simulink model "extra_simulink"  (R2021a)
settings: Solver=VariableStepAuto  StartTime=0.0  StopTime=10  MaxStep=1e-4  RelTol=1e-3
undefined symbols (not defined in the file): b1, b2, b3, F_1, F_2, F_3, k1, k2, k3, m1, m2, m3, time_F_1, time_F_2, time_F_3, x1_0, x2_0, x3_0
settings Model: Creator=SPb19  LastModifiedBy=SPb19

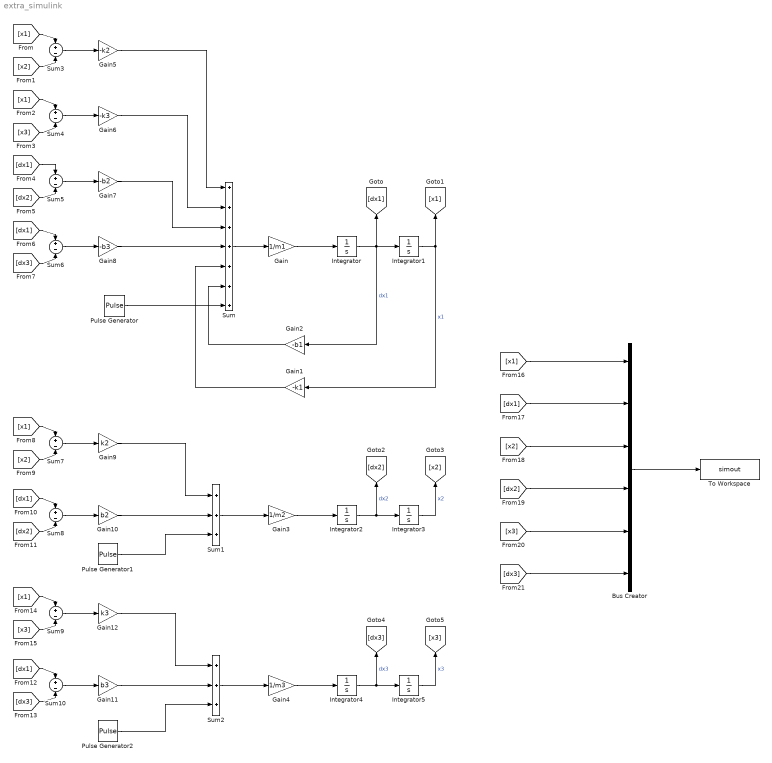
== system extra_simulink ==
  Bus Creator : BusCreator  Inputs=6
  Gain : Gain  Gain=1/m1
  Gain1 : Gain  Gain=-k1
  Gain10 : Gain  Gain=b2
  Gain11 : Gain  Gain=b3
  Gain12 : Gain  Gain=k3
  Gain2 : Gain  Gain=-b1
  Gain3 : Gain  Gain=1/m2
  Gain4 : Gain  Gain=1/m3
  Gain5 : Gain  Gain=-k2
  Gain6 : Gain  Gain=-k3
  Gain7 : Gain  Gain=-b2
  Gain8 : Gain  Gain=-b3
  Gain9 : Gain  Gain=k2
  Integrator : Integrator
  Integrator1 : Integrator  InitialCondition=x1_0
  Integrator2 : Integrator
  Integrator3 : Integrator  InitialCondition=x2_0
  Integrator4 : Integrator
  Integrator5 : Integrator  InitialCondition=x3_0
  Pulse Generator : DiscretePulseGenerator  PulseType=Time based  Amplitude=F_1  Period=t + 10  PulseWidth=100 * time_F_1 / (t + 10)
  Pulse Generator1 : DiscretePulseGenerator  PulseType=Time based  Amplitude=F_2  Period=t + 10  PulseWidth=100 * time_F_2 / (t + 10)
  Pulse Generator2 : DiscretePulseGenerator  PulseType=Time based  Amplitude=F_3  Period=t + 10  PulseWidth=100 * time_F_3 / (t + 10)
  Sum : Sum  Inputs=+++++++
  Sum1 : Sum  Inputs=+++
  Sum{3..10} (8 alike) : Sum  Inputs=+-
  Sum2 : Sum  Inputs=+++
  To Workspace : ToWorkspace  VariableName=simout  SaveFormat=Timeseries  SampleTime=-1
  wires:
  Gain/1 -> Integrator/1
  Integrator/1 -> [dx1], Gain2/1, Integrator1/1  "dx1"
  Sum/1 -> Gain/1
  Integrator1/1 -> [x1], Gain1/1  "x1"
  Gain1/1 -> Sum/5
  Gain2/1 -> Sum/6
  Sum1/1 -> Gain3/1
  Integrator3/1 -> [x2]  "x2"
  Integrator2/1 -> [dx2], Integrator3/1  "dx2"
  Gain3/1 -> Integrator2/1
  Integrator4/1 -> [dx3], Integrator5/1  "dx3"
  Gain4/1 -> Integrator4/1
  Integrator5/1 -> [x3]  "x3"
  Sum2/1 -> Gain4/1
  [x1] -> Sum3/1
  [x2] -> Sum3/2
  Sum3/1 -> Gain5/1
  Gain5/1 -> Sum/1
  Sum4/1 -> Gain6/1
  [x1] -> Sum4/1
  [x3] -> Sum4/2
  Gain6/1 -> Sum/2
  [dx2] -> Sum5/2
  [dx1] -> Sum5/1
  Sum5/1 -> Gain7/1
  Gain7/1 -> Sum/3
  Sum6/1 -> Gain8/1
  [dx1] -> Sum6/1
  [dx3] -> Sum6/2
  Gain8/1 -> Sum/4
  Sum7/1 -> Gain9/1
  [x1] -> Sum7/1
  [x2] -> Sum7/2
  Gain9/1 -> Sum1/1
  Sum8/1 -> Gain10/1
  [dx1] -> Sum8/1
  [dx2] -> Sum8/2
  Gain10/1 -> Sum1/2
  [x3] -> Sum9/2
  [dx3] -> Sum10/2
  [dx1] -> Sum10/1
  Sum10/1 -> Gain11/1
  Sum9/1 -> Gain12/1
  [x1] -> Sum9/1
  Gain12/1 -> Sum2/1
  Gain11/1 -> Sum2/2
  [x1] -> Bus Creator/1
  [dx1] -> Bus Creator/2
  [dx3] -> Bus Creator/6
  [x3] -> Bus Creator/5
  [dx2] -> Bus Creator/4
  [x2] -> Bus Creator/3
  Bus Creator/1 -> To Workspace/1
  Pulse Generator/1 -> Sum/7
  Pulse Generator1/1 -> Sum1/3
  Pulse Generator2/1 -> Sum2/3
